simulink model "apparent_temp"  (R2020b)
settings: Solver=VariableStepAuto  StartTime=0.0  StopTime=10.0  RelTol=1e-3
settings Model: Creator=Litao  LastModifiedBy=Litao

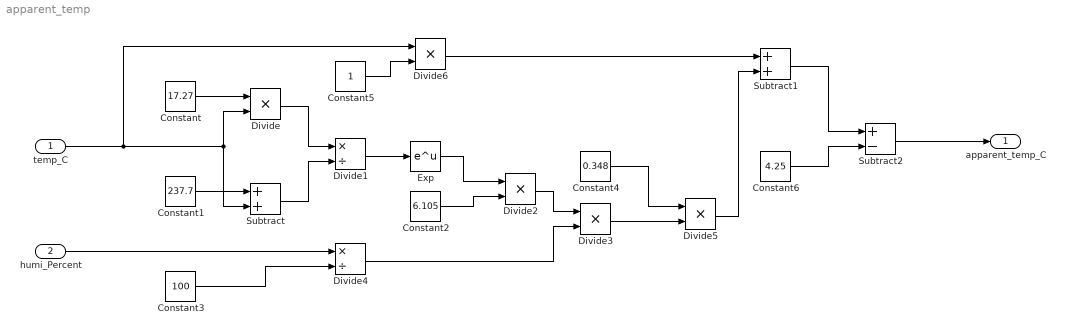
== system apparent_temp ==
  temp_C : Inport  OutDataTypeStr=double
  humi_Percent : Inport  Port=2  OutDataTypeStr=double
  Constant : Constant  Value=17.27
  Constant1 : Constant  Value=237.7
  Constant2 : Constant  Value=6.105
  Constant3 : Constant  Value=100
  Constant4 : Constant  Value=0.348
  Constant5 : Constant
  Constant6 : Constant  Value=4.25
  Divide{,2..3,5..6} (5 alike) : Product  Inputs=**
  Divide1 : Product  Inputs=*/
  Divide4 : Product  Inputs=*/
  Exp : Math  SaturateOnIntegerOverflow=on
  Subtract : Sum
  Subtract1 : Sum
  Subtract2 : Sum  Inputs=+-
  apparent_temp_C : Outport
  wires:
  Constant1/1 -> Subtract/1
  temp_C/1 -> Divide6/1, Subtract/2, Divide/2
  Constant/1 -> Divide/1
  Divide/1 -> Divide1/1
  Subtract/1 -> Divide1/2
  Divide1/1 -> Exp/1
  Exp/1 -> Divide2/1
  Constant2/1 -> Divide2/2
  humi_Percent/1 -> Divide4/1
  Constant3/1 -> Divide4/2
  Divide4/1 -> Divide3/2
  Divide2/1 -> Divide3/1
  Divide3/1 -> Divide5/2
  Constant4/1 -> Divide5/1
  Divide5/1 -> Subtract1/2
  Subtract1/1 -> Subtract2/1
  Constant6/1 -> Subtract2/2
  Subtract2/1 -> apparent_temp_C/1
  Constant5/1 -> Divide6/2
  Divide6/1 -> Subtract1/1
